simulink model "mixedmanchester"  (Simulink 5.1)
settings: Solver=FixedStepDiscrete  SolverMode=SingleTasking  StartTime=0.0  StopTime=50000  RelTol=1e-3
undefined symbols (not defined in the file or in its folder): sigbuilder_block
libraries: fixpt_lib_4 x3, simulink x2, dspsigops x2, dspsrcs4 x1, modelsimlib x1
settings Model: Creator=adowd  LastModifiedBy=lluo  ExtModeAutoUpdateStatusClock=off  BooleanDataType=on  ProdHWDeviceType=Microprocessor  RTWOptions="-aEnforceIntegerDowncast=1 -aExtMode=0 -aExtModeTesting=0 -aFoldNonRolledExpr=1 -aForceParamTrailComments=0 -aGenerateComments=1 -aGenerateReport=0 -aIgnoreCustomStorageClasses=1 -aIncDataTypeInIds=0 -aIncHierarchyInIds=0 -aInlineInvariantSignals=0 -aInlinedPrmAccess=\"Literals\" -aLocalBlockOutputs=1 -aLogVarNameModifier=\"rt_\" -aMaxRTWIdLen=31 -aPrefixModelToSubsysFcnNames=1 -aRTWVerbose=1 -aRollThreshold=5 -aShowEliminatedStatements=0"

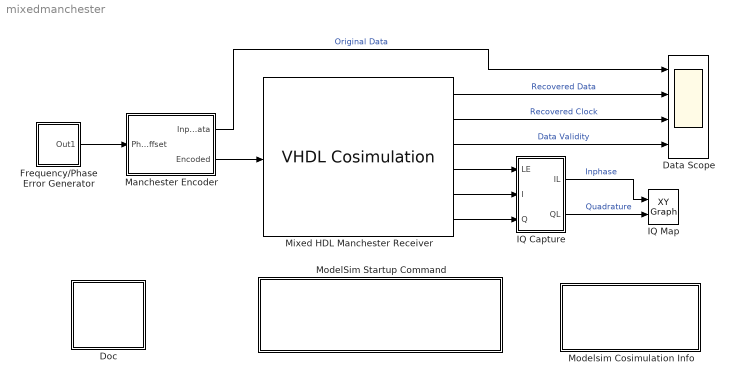
== system mixedmanchester ==
  Data Scope : Scope  NumInputPorts=4
      settings: TimeRange=3000  YMin=-1~-1~-1~0.95  YMax=2~2~2~1.05
  Doc : Subsystem
      settings: OpenFcn=web(fullfile(matlabroot,'toolbox','modelsim','modelsimdemos','html','manchesterreceiverdemo.html'))
      mask Type: VHDL Manchester Receiver Demo Info
      mask Display: disp('Info')
  Frequency/Phase Error Generator : Subsystem
  IQ Capture : Subsystem
  IQ Map : simulink/Sinks/XY Graph  xmin=0  xmax=16  ymin=0  ymax=16  st=-1
  Manchester Encoder : Subsystem
  Mixed HDL Manchester Receiver : modelsimlib/VHDL Cosimulation  idxCellArray={'/manchester/samp', 'in', '/manchester/data', 'out', '/manchester/dclk', 'out', '/manchester/dvalid', 'out', '/manchester/sync_i', 'out', '/manchester/isum_i', 'out', '/manchester/qsum_i', 'out', '/manchester/clk', 'rclk'}  Tso=-1  tclBefore=force /manchester/enable 1 0; force sim:/manchester/reset 1 0, 0 1000 ns  tclAfter="echo \"done\""  hostName='modelsim_comp'  portNumber=4442  modelSimRunning=on  sharedMemory=on
  ModelSim Startup Command : Subsystem
      settings: OpenFcn=vsim('tclstart',mixedmanchestercmds)
      mask Type: VHDL Manchester Receiver Demo Info
      mask Display: disp(['vsim(''tclstart'',mixedmanchestercmds)', char(10),'%', 'Double click to launch a new ModelSim'])
  Modelsim Cosimulation Info : Subsystem
      mask Type: Verilog Manchester Receiver Demo Info
      mask Display: disp('Mixed HDL Manchester\nEncoder Simulation\nInformation')
  wires:
  Manchester Encoder/2(Encoded) -> Mixed HDL Manchester Receiver/1
  Mixed HDL Manchester Receiver/3 -> Data Scope/4  "Data Validity"
  Frequency/Phase Error Generator/1(Out1) -> Manchester Encoder/1(Phase  Offset)
  Mixed HDL Manchester Receiver/2 -> Data Scope/3  "Recovered Clock"
  Manchester Encoder/1(Input Data) -> Data Scope/1  "Original Data"
  Mixed HDL Manchester Receiver/1 -> Data Scope/2  "Recovered Data"
  Mixed HDL Manchester Receiver/4 -> IQ Capture/1(LE)
  Mixed HDL Manchester Receiver/6 -> IQ Capture/3(Q)
  Mixed HDL Manchester Receiver/5 -> IQ Capture/2(I)
  IQ Capture/1(IL) -> IQ Map/1  "Inphase"
  IQ Capture/2(QL) -> IQ Map/2  "Quadrature"

== system mixedmanchester/Doc ==

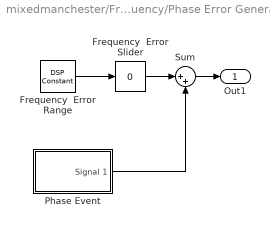
== system mixedmanchester/Frequency/Phase Error Generator ==
  Frequency  Error Range : dspsrcs4/DSP Constant  Value=1/128  SampleMode=Discrete  discreteOutput=Sample-based  continuousOutput=Sample-based  sampTime=10  framePeriod=2  dataType=Inherit from 'Constant value'  wordLen=16  udDataType=sfix(16)  fracBitsMode=Best precision  numFracBits=15  InterpretAs1D=-inf  Ts=-inf  FramebasedOutput=-inf
  Frequency  Error Slider : simulink/Math Operations/Slider Gain  low=-1  gain=0  high=1
  Phase Event : Subsystem  Tag=STV Subsys  StartFcn=sigbuilder_block('start');  StopFcn=sigbuilder_block('stop');  ClipboardFcn=sigbuilder_block('clipboard');  mask(Sigbuilder block){}
      mask help: Sigbuilder GUI
      mask init:
      | if ~strcmp(get_param(bdroot(gcb),'SimulationStatus'),'stopped') tuvar = sigbuilder_block('maskInit'); end
      settings: CopyFcn=sigbuilder_block('copy');  DeleteFcn=sigbuilder_block('delete');  ModelCloseFcn=sigbuilder_block('modelClose');  PreSaveFcn=sigbuilder_block('preSave');  NameChangeFcn=sigbuilder_block('namechange');  OpenFcn=sigbuilder_block('open',[90.75 75 522.75 365.25 ]);  CloseFcn=sigbuilder_block('close');
      mask Display: plot(0,0,100,100,[10,10,40,40,10],[80,20,20,80,80],[40,10],[50,50], [40,27,10],[65,72,56],[40,25,25,10],[28,28,43,43]);
  Sum : Sum  Inputs=|++  SaturateOnIntegerOverflow=on
  Out1 : Outport
  wires:
  Phase Event/1(Signal 1) -> Sum/2
  Frequency  Error Range/1 -> Frequency  Error Slider/1
  Frequency  Error Slider/1 -> Sum/1
  Sum/1 -> Out1/1

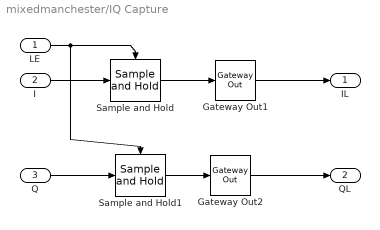
== system mixedmanchester/IQ Capture ==
  LE : Inport
  I : Inport  Port=2
  Q : Inport  Port=3
  Gateway Out1 : fixpt_lib_4/Data Type/Gateway Out  OutRealWorld=Real World Value  OutBuiltInType=double  RndMeth=Nearest  DoSatur=off
  Gateway Out2 : fixpt_lib_4/Data Type/Gateway Out  OutRealWorld=Real World Value  OutBuiltInType=double  RndMeth=Nearest  DoSatur=off
  Sample and Hold : dspsigops/Sample and Hold  trig=Rising edge  initCond=0
  Sample and Hold1 : dspsigops/Sample and Hold  trig=Rising edge  initCond=0
  IL : Outport
  QL : Outport  Port=2
  wires:
  LE/1 -> Sample and Hold/Trigger, Sample and Hold1/Trigger
  Sample and Hold/1 -> Gateway Out1/1
  Sample and Hold1/1 -> Gateway Out2/1
  Gateway Out1/1 -> IL/1
  Gateway Out2/1 -> QL/1
  I/1 -> Sample and Hold/1
  Q/1 -> Sample and Hold1/1

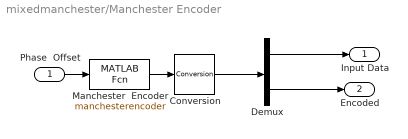
== system mixedmanchester/Manchester Encoder ==
  Phase  Offset : Inport
  Conversion : fixpt_lib_4/Data Type/Conversion  ConvertRealWorld=Real World Value  OutputDataTypeScalingMode=Specify via dialog  OutDataType=ufix(1)  OutScaling=1  DoSatur=off
  Demux : Demux  Outputs=2
  Manchester  Encoder : MATLABFcn  MATLABFcn=manchesterencoder
  Input Data : Outport
  Encoded : Outport  Port=2
  wires:
  Manchester  Encoder/1 -> Conversion/1
  Conversion/1 -> Demux/1
  Demux/1 -> Input Data/1
  Phase  Offset/1 -> Manchester  Encoder/1
  Demux/2 -> Encoded/1

== system mixedmanchester/ModelSim Startup Command ==

== system mixedmanchester/Modelsim Cosimulation Info ==
  note: Manchester Recevier
      |
      |
      | Manchester encoding is a simple modulation scheme which converts baseband digital
      | data into an encoded waveform with no DC component.  The most widely known
      | application of this technique is Ethernet.
      |
      | This model simulates a pure-digital receiver of Manchester encoded data.  The receiver is
      | implemented in VHDL/Verilog. The receiver uses a simple DLL clock recovery mechanism,
      | which requires multiple cycles to lock with the incoming data stream.  The performance of
      | the receiver is explored by applying phase and frequency errors to a randomly generated
      | steam of bits that is encoded using a simple MATLAB function: manchesterencoder().
      |
      | The actual VHDL/Verilog code will run in ModelSim using the cosimulation block
      | called "Mixed HDL Manchester Receiver"

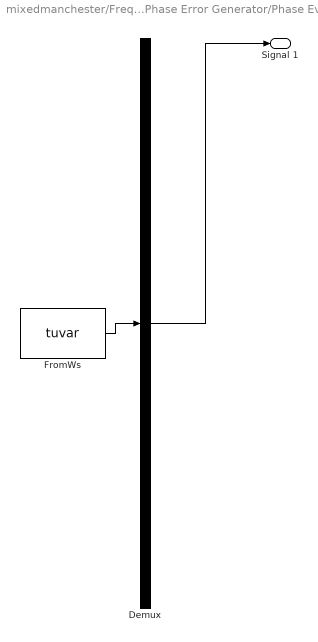
== system mixedmanchester/Frequency/Phase Error Generator/Phase Event ==
  Demux : Demux  Tag=STV Demux  Outputs=1
  FromWs : FromWorkspace  Tag=STV FromWs  VariableName=tuvar  SampleTime=10  OutputAfterFinalValue=Holding final value  SigBuilderData=DataTag0
      SigBuilderData=|
      | channels.label = 'Signal 1'
      | channels.allXData = {[0 20020 20020 20570 20570 30000]}
      | channels.allYData = {[-0.0005 -0.0005 0.0794 0.0794 0 0]}
      | common.afterFinalStr = 'Hold final value'
      | common.sampleTime = 10
      | dataSet.timeRange = [0 30000]
      | dataSet.name = 'Group 1'
  Signal 1 : Outport  Tag=STV Outport
  wires:
  Demux/1 -> Signal 1/1
  FromWs/1 -> Demux/1
